simulink model "wolnozmienny_kwantyzacja"  (R2017b)
settings: Solver=FixedStepDiscrete  StartTime=0.0  StopTime=0.0  RelTol=1e-3
undefined symbols (not defined in the file): H, W
libraries: CPOiS_SourcesSinks x6, CPOiS_DataManipulation x2
settings Model: Creator=alis  LastModifiedBy=alis

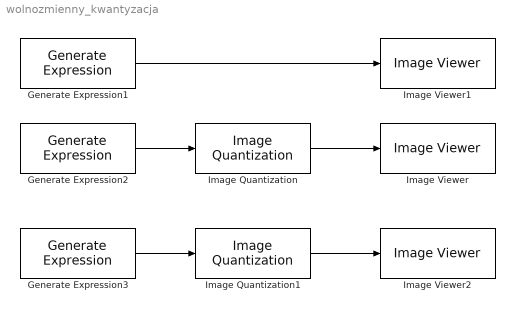
== system wolnozmienny_kwantyzacja ==
  Generate Expression1 : CPOiS_SourcesSinks/Generate Expression  Width=256  Height=256  Expression=W/2+H/2
      settings: SourceProductName=CPOiS - Digital image and signal processing
  Generate Expression2 : CPOiS_SourcesSinks/Generate Expression  Width=256  Height=256  Expression=W/2+H/2
      settings: SourceProductName=CPOiS - Digital image and signal processing
  Generate Expression3 : CPOiS_SourcesSinks/Generate Expression  Width=256  Height=256  Expression=W/2+H/2
      settings: SourceProductName=CPOiS - Digital image and signal processing
  Image Quantization : CPOiS_DataManipulation/Image Quantization  LevelsNum=5
      settings: SourceProductName=CPOiS - Digital image and signal processing
  Image Quantization1 : CPOiS_DataManipulation/Image Quantization  LevelsNum=2
      settings: SourceProductName=CPOiS - Digital image and signal processing
  Image Viewer : CPOiS_SourcesSinks/Image Viewer
      settings: SourceProductName=CPOiS - Digital image and signal processing
  Image Viewer1 : CPOiS_SourcesSinks/Image Viewer
      settings: SourceProductName=CPOiS - Digital image and signal processing
  Image Viewer2 : CPOiS_SourcesSinks/Image Viewer
      settings: SourceProductName=CPOiS - Digital image and signal processing
  wires:
  Generate Expression2/1 -> Image Quantization/1
  Image Quantization/1 -> Image Viewer/1
  Generate Expression1/1 -> Image Viewer1/1
  Generate Expression3/1 -> Image Quantization1/1
  Image Quantization1/1 -> Image Viewer2/1
